simulink model "Dyn_model"  (R2024b)
settings: Solver=VariableStepAuto  StartTime=0.0  StopTime=10.0  RelTol=1e-3
values from neighbouring files (symbols this model uses):
  A = [A_top; A_bottom]    [Dynamic_model.m]    (also in MonteCarlo.m = [zeros(n), eye(n); -Ms\Ks, -Ms\Cs])
  Bce = [Bc, E]    [Dynamic_model.m]
  C = [C_top; C_bottom]    [Dynamic_model.m]
  Dcf = [Dc, F]    [Dynamic_model.m]
settings Model: Creator=Arghya  LastModifiedBy=Arghya

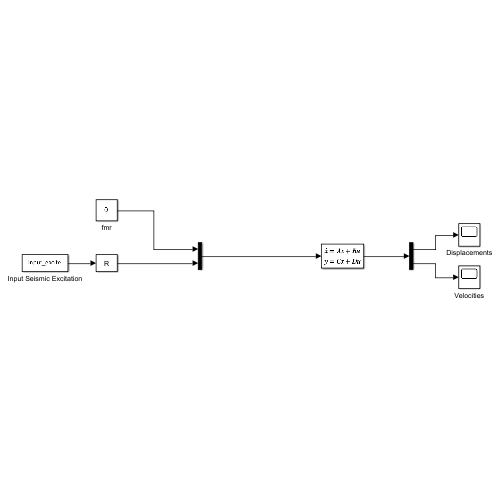
[thumbnail: Simulink's stored preview of the top-level diagram]
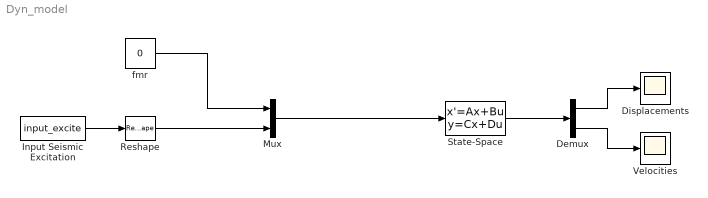
== system Dyn_model ==
  Demux : Demux  Outputs=2
  Displacements : Scope
  Input Seismic Excitation : FromWorkspace  VariableName=input_excite  OutputAfterFinalValue=Setting to zero
  Mux : Mux  Inputs=2
  Reshape : Reshape  OutputDimensionality=Customize
  State-Space : StateSpace  A=A  B=Bce  C=C  D=Dcf  InitialCondition=0  ContinuousStateAttributes="\"Building\""
  Velocities : Scope
  fmr : Constant  Value=0  SampleTime=0.002
  wires:
  State-Space/1 -> Demux/1
  fmr/1 -> Mux/1
  Demux/2 -> Velocities/1
  Demux/1 -> Displacements/1
  Input Seismic Excitation/1 -> Reshape/1
  Reshape/1 -> Mux/2
  Mux/1 -> State-Space/1
